simulink model "SimulationTest"  (R2025a)
settings: Solver=ode45  StartTime=0.0  StopTime=2000  FixedStep=0.01  MaxStep=0.01  MinStep=0.001  RelTol=1e-3
model workspace (MAT data in the model file):
  L = 0.25
  R = 0.05
libraries: simulink x5
settings Model: PacingRate=1000  Creator=levirogalla  LastModifiedBy=levirogalla

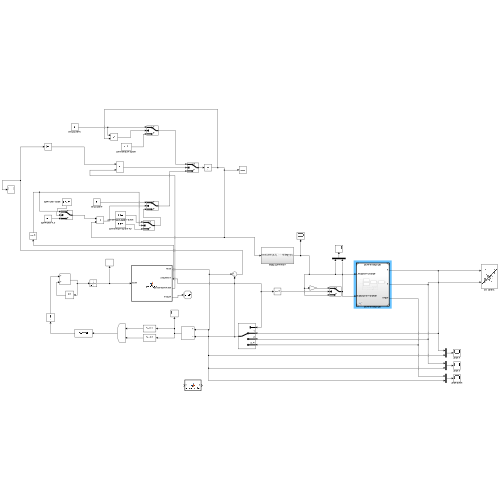
[thumbnail: Simulink's stored preview of the top-level diagram]
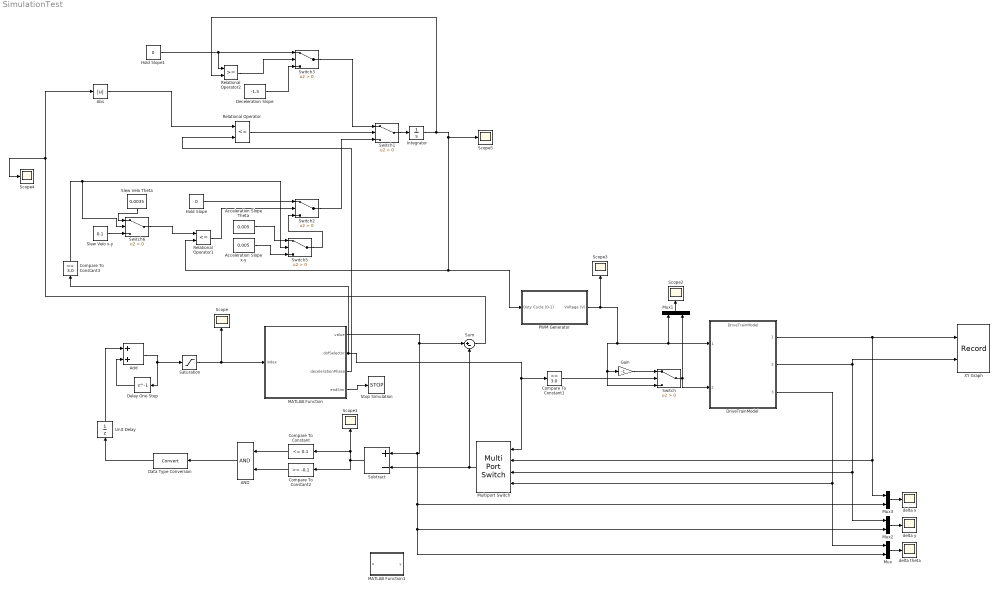
== system SimulationTest ==
  AND : Logic  IconShape=distinctive  AllPortsSameDT=off  OutDataTypeStr=boolean
  Abs : Abs  SaturateOnIntegerOverflow=off
  Acceleration Slope Theta : Constant  Value=0.005
  Acceleration Slope x-y : Constant  Value=0.005
  Add : Sum
  Compare To Constant : simulink/Logic and Bit Operations/Compare To Constant  relop=<=  const=0.1  OutDataTypeStr=boolean
  Compare To Constant1 : simulink/Logic and Bit Operations/Compare To Constant  relop===  const=3.0  OutDataTypeStr=boolean
  Compare To Constant2 : simulink/Logic and Bit Operations/Compare To Constant  relop=>=  const=-0.1  OutDataTypeStr=boolean
  Compare To Constant3 : simulink/Logic and Bit Operations/Compare To Constant  relop===  const=3.0  OutDataTypeStr=boolean
  Data Type Conversion : DataTypeConversion  SaturateOnIntegerOverflow=off  RndMeth=Floor
  Deceleration Slope : Constant  Value=-1.5
  Delay One Step : Delay  DelayLength=1
  DriveTrainModel : ModelReference  ModelNameDialog=DriveTrainModel.slx  SimulationMode=Normal  ModelReferenceVersion=1.8
  Gain : Gain  Gain=-1
  Hold Slope : Constant  Value=0
  Hold Slope1 : Constant  Value=0
  Integrator : Integrator
  MATLAB Function : MATLAB Function  TreatAsAtomicUnit=on
  MATLAB Function1 : MATLAB Function  TreatAsAtomicUnit=on
  Multiport Switch : MultiPortSwitch  SaturateOnIntegerOverflow=off  InputSameDT=off
  Mux{,1..3} (4 alike) : Mux  Inputs=2
  PWM Generator : Subsystem
  Relational Operator : RelationalOperator  Operator=<=  OutDataTypeStr=boolean  RndMeth=Simplest  InputSameDT=off
  Relational Operator1 : RelationalOperator  Operator=<=  OutDataTypeStr=boolean  RndMeth=Simplest  InputSameDT=off
  Relational Operator2 : RelationalOperator  OutDataTypeStr=boolean  RndMeth=Simplest  InputSameDT=off
  Saturation : Saturate  UpperLimit=5  LowerLimit=0  LinearizeAsGain=off
  Scope{,1..5} (6 alike) : Scope
      Scope settings: ActiveDisplayYMinimum=-0.125  ActiveDisplayYMaximum=1.125
      Scope1 settings: ActiveDisplayYMinimum=-22.01338  ActiveDisplayYMaximum=19.1126  DataLoggingVariableName=ScopeData2
      Scope2 settings: ActiveDisplayYMinimum=-3.75  ActiveDisplayYMaximum=3.75
      Scope3 settings: ActiveDisplayYMinimum=-1.5  ActiveDisplayYMaximum=13.5  DataLoggingVariableName=ScopeData2
      Scope4 settings: ActiveDisplayYMinimum=-19.18386  ActiveDisplayYMaximum=19.05022  DataLoggingVariableName=ScopeData3
      Scope5 settings: ActiveDisplayYMinimum=-0.0125  ActiveDisplayYMaximum=0.1125  DataLoggingVariableName=ScopeData4
  Slew Velo Theta : Constant  Value=0.0035
  Slew Velo x-y : Constant  Value=0.1
  Stop Simulation : Stop
  Subtract : Sum  Inputs=+-
  Sum : Sum  Inputs=|+-
  Switch{,1..3,5..6} (6 alike) : Switch  Criteria=u2 > Threshold  SaturateOnIntegerOverflow=off  InputSameDT=off
  Unit Delay : UnitDelay  SampleTime=-1  HasFrameUpgradeWarning=on
  XY Graph : Record  NumPorts=2.0  FileSettingsInternal="{\"entries\":[{\"content\":{\"excelSettings\":{\"content\":{},\"type\":\"Streamout.ExcelSettings\"},\"parquetSettings\":{\"content\":{},\"type\":\"Streamout.ParquetSettings\"}},\"type\":\"Streamout.FileSettingStorage\",\"uuid\":\"\"}],\"packageUris\":[\"http:\\/\\/schema.mathworks.com\\/mf0\\/streamout_blocks\\/R2020a\"],\"version\":\"1.0\"}"  FrameSettings=[0, 0]  Layout=[1 1]  SignalsInternal="{\"entries\":[{\"content\":{\"signals\":[{\"content\":{\"blockPath\":[],\"dimensions\":[1],\"domain\":\"\",\"lineColor\":\"#a2142f\",\"plots\":[ 1 ],\"port\":1,\"sid\":[\"\"],\"signalID\":1,\"signalName\":\"DriveTrainModel:1\"},\"type\":\"RecordBlkView.Signal\",\"uuid\":\"\"},{\"content\":{\"blockPath\":[],\"dimensions\":[1],\"domain\":\"\",\"lineColor\":\"#139fff\",\"plots\":[ 1 ],\"port\":2,\"sid\":[\"\"],\"signalID\":2,\"signalName\":\"DriveTrainModel:2\"},\"type\":\"RecordBlkView.Signal\",\"uuid\":\"\"}]},\"type\":\"RecordBlkView.InputSignals\",\"uuid\":\"\"}],\"packageUris\":[\"http:\\/\\/schema.mathworks.com\\/mf0\\/streamout_blocks\\/R2020a\"],\"version\":\"1.0\"}"  VisualizationBindings="{\"xyplotplugin\":{\"info\":[{\"series\":[{\"bindingParametersList\":[{\"parameter\":\"X-Axis\",\"signalID\":1,\"signalName\":\"DriveTrainModel:1\"},{\"parameter\":\"Y-Axis\",\"signalID\":2,\"signalName\":\"DriveTrainModel:2\"}],\"seriesID\":0}],\"subplotID\":1}]}}"  CompatibilityTag=XY
  delta theta : Scope
      settings: ActiveDisplayYMinimum=-12.11497  ActiveDisplayYMaximum=15.46071
  delta x : Scope
      settings: ActiveDisplayYMinimum=-13.38343  ActiveDisplayYMaximum=19.45083  DataLoggingVariableName=ScopeData2
  delta y : Scope
      settings: ActiveDisplayYMinimum=-13.54734  ActiveDisplayYMaximum=18.17193  DataLoggingVariableName=ScopeData3
  wires:
  DriveTrainModel/2 -> XY Graph/2, Mux2/1, Multiport Switch/3
  DriveTrainModel/1 -> Multiport Switch/2, Mux3/1, XY Graph/1
  DriveTrainModel/3 -> Mux/1, Multiport Switch/4
  MATLAB Function/1(value) -> Sum/1, Mux/2, Mux2/2, Mux3/2, Subtract/1
  Multiport Switch/1 -> Subtract/2, Sum/2
  Add/1 -> Delay One Step/1, Saturation/1
  Delay One Step/1 -> Add/2
  MATLAB Function/2(dofSelector) -> Multiport Switch/1, Compare To Constant1/1, Compare To Constant3/1
  Subtract/1 -> Compare To Constant2/1, Scope1/1, Compare To Constant/1
  Data Type Conversion/1 -> Unit Delay/1
  Saturation/1 -> MATLAB Function/1(index), Scope/1
  Unit Delay/1 -> Add/1
  Mux1/1 -> Scope2/1
  Compare To Constant2/1 -> AND/2
  Compare To Constant/1 -> AND/1
  AND/1 -> Data Type Conversion/1
  Compare To Constant1/1 -> Switch/2
  Switch/1 -> DriveTrainModel/2, Mux1/2
  Gain/1 -> Switch/1
  Mux/1 -> delta theta/1
  Mux3/1 -> delta x/1
  Mux2/1 -> delta y/1
  MATLAB Function/4(endSim) -> Stop Simulation/1
  PWM Generator/1(Voltage (V)) -> DriveTrainModel/1, Mux1/1, Switch/3, Gain/1, Scope3/1
  Sum/1 -> Abs/1, Scope4/1
  Relational Operator2/1 -> Switch3/2
  Deceleration Slope/1 -> Switch3/3
  Hold Slope/1 -> Switch2/1
  Hold Slope1/1 -> Relational Operator2/1, Switch3/1
  Switch3/1 -> Switch1/1
  Relational Operator/1 -> Switch1/2
  Acceleration Slope x-y/1 -> Switch5/3
  Switch1/1 -> Integrator/1
  Switch2/1 -> Switch1/3
  Relational Operator1/1 -> Switch2/2
  Integrator/1 -> Relational Operator2/2, Scope5/1, PWM Generator/1(Duty Cycle (0-1)), Relational Operator1/2
  Compare To Constant3/1 -> Switch5/2, Switch6/2
  MATLAB Function/3(decelerationPhase) -> Relational Operator/2
  Acceleration Slope Theta/1 -> Switch5/1
  Switch5/1 -> Switch2/3
  Slew Velo x-y/1 -> Switch6/3
  Slew Velo Theta/1 -> Switch6/1
  Switch6/1 -> Relational Operator1/1
  Abs/1 -> Relational Operator/1

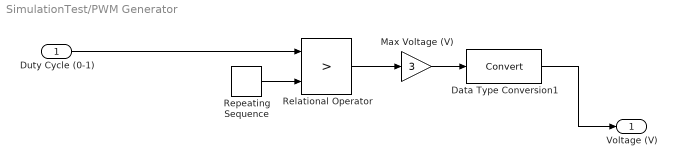
== system SimulationTest/PWM Generator ==
  Duty Cycle (0-1) : Inport
  Data Type Conversion1 : DataTypeConversion  SaturateOnIntegerOverflow=off  RndMeth=Floor
  Max Voltage (V) : Gain  Gain=3
  Relational Operator : RelationalOperator  Operator=>  OutDataTypeStr=boolean  RndMeth=Simplest  InputSameDT=off
  Repeating Sequence : simulink/Sources/Repeating Sequence  rep_seq_t=[0 0.1]  rep_seq_y=[0 1]
  Voltage (V) : Outport
  wires:
  Data Type Conversion1/1 -> Voltage (V)/1
  Repeating Sequence/1 -> Relational Operator/2
  Relational Operator/1 -> Max Voltage (V)/1
  Max Voltage (V)/1 -> Data Type Conversion1/1
  Duty Cycle (0-1)/1 -> Relational Operator/1

== matlab function SimulationTest/MATLAB Function1 ==
  data: u input; y output
function y = phaseChecker(u)

y = u;

== matlab function SimulationTest/MATLAB Function ==
  data: value output; dofSelector output; decelerationPhase output; index input; endSim output
function [value, dofSelector, decelerationPhase, endSim] = pathSignal(index)
% Returns path values and a signal to stop simulation when out of bounds

% Define the path matrix
pathMatrix = [15, 1, 4;
             -pi/2, 3, 1;
             -10.1, 2, 3.8;
             -pi, 3, 1;
              6.9, 1, 3];

% Get the size of the path
N = size(pathMatrix, 1);

% Initialize outputs
value = 0;
dofSelector = 1;
decelerationPhase = 0;
endSim = false;

% Check if index is within bounds
if index + 1 <= N
    value = pathMatrix(index + 1, 1);
    dofSelector = pathMatrix(index + 1, 2);
    decelerationPhase = pathMatrix(index + 1, 3);
else
    endSim = true;  % signal to stop the simulation
end
